simulink model "rst_auto_reg_coupled_tanks_2018b"  (R2018b)
settings: Solver=ode45  StartTime=0.0  StopTime=1000  RelTol=1e-3
InitFcn:
  | g = 981
  | Km = 3.3
  | Ao1 = 0.17
  | At1 = 15.5528
  | Ao2 = 0.17
  | At2 = 15.5528
  | Ta = 0.1
  | Ts = 50
  | ep = 0.7
libraries: dspinverses x2
settings Model: Creator=root  LastModifiedBy=root
settings DataIOCC: SaveFormat=StructureWithTime
settings OptimizationCC: LifeSpan=inf
settings DebuggingCC: LibraryContextMissingDiagnostic=none  SFExecutionAtInitializationDiag=none
settings HardwareCC: ProdBitPerSizeT=32  ProdBitPerPtrDiffT=32  ProdWordSize=32  ProdHWDeviceType=Specified
settings CodeAppCC: StateflowObjectComments=on

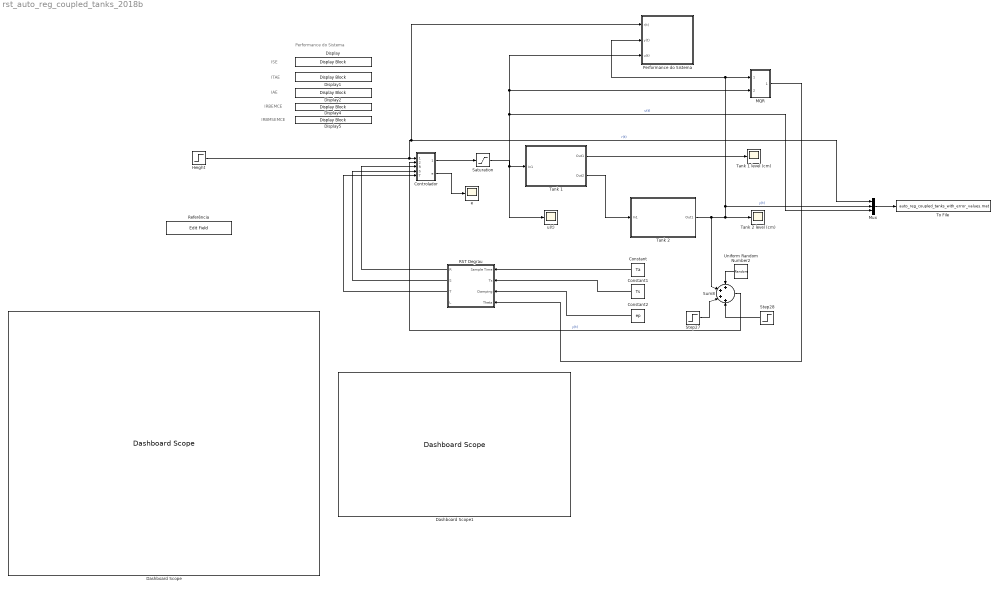
== system rst_auto_reg_coupled_tanks_2018b ==
  note: IAE
  note: IRBEMCE
  note: ISE
  note: ITAE
  note: IRBMSEMCE
  note: Performance do Sistema
  Constant : Constant  Value=Ta
  Constant1 : Constant  Value=Ts
  Constant2 : Constant  Value=ep
  Controlador : Subsystem
  Dashboard Scope : DashboardScope  WebBlockId=688
  Dashboard Scope1 : DashboardScope  WebBlockId=689
  Display : DisplayBlock  WebBlockId=787  LabelPosition=Hide
  Display1 : DisplayBlock  WebBlockId=788  LabelPosition=Hide
  Display2 : DisplayBlock  WebBlockId=789  LabelPosition=Hide
  Display4 : DisplayBlock  WebBlockId=790  LabelPosition=Hide
  Display5 : DisplayBlock  WebBlockId=791  LabelPosition=Hide
  Height : Step  Time=0  After=15  SampleTime=0
  MQR : Subsystem
  Mux : Mux  Inputs=3
  Performance do Sistema : Subsystem
  RST Degrau : Subsystem
  Referência : EditField  WebBlockId=683  LabelPosition=Hide  Alignment=Center
  Saturation : Saturate  UpperLimit=12  LowerLimit=-12
  Step27 : Step  Time=150  SampleTime=0
  Step28 : Step  Time=151  After=-1  SampleTime=0
  Sum8 : Sum  Inputs=++++
  Tank 1 : Subsystem
  "Tank 1 level (cm) " : Scope
  Tank 2 : Subsystem
  "Tank 2 level (cm) " : Scope
  To File : ToFile  Filename=auto_reg_coupled_tanks_with_error_values.mat
  Uniform Random Number2 : UniformRandomNumber  Minimum=-0.01  Maximum=0.01  SampleTime=0
  e : Scope
  u(t) : Scope
  wires:
  Constant2/1 -> RST Degrau/3(Damping)
  Constant/1 -> RST Degrau/1(Sample Time)
  Constant1/1 -> RST Degrau/2(Ts)
  MQR/1("Theta(t) ") -> RST Degrau/4(Theta)
  Tank 1/1(Out1) -> "Tank 1 level (cm) "/1
  Tank 1/2(Out2) -> Tank 2/1(In1)
  RST Degrau/1(R) -> Controlador/3(R)
  RST Degrau/2(S) -> Controlador/4(S)
  RST Degrau/3(T) -> Controlador/5(T)
  Controlador/1(u(t)) -> Saturation/1
  Controlador/2("e ") -> e/1
  Step27/1 -> Sum8/3
  Step28/1 -> Sum8/4
  Uniform Random Number2/1 -> Sum8/1
  Sum8/1 -> Controlador/2(y(t))  "y(t)"
  Mux/1 -> To File/1
  Saturation/1 -> u(t)/1, Mux/3, Performance do Sistema/3(u(t)), MQR/2("u(t) "), Tank 1/1(In1)  "u(t)"
  Tank 2/1(Out1) -> Sum8/2, Mux/2, Performance do Sistema/2(y(t)), MQR/1(y(t)), "Tank 2 level (cm) "/1  "y(t)"
  Height/1 -> Performance do Sistema/1(r(t)), Mux/1, Controlador/1(r(t))  "r(t)"

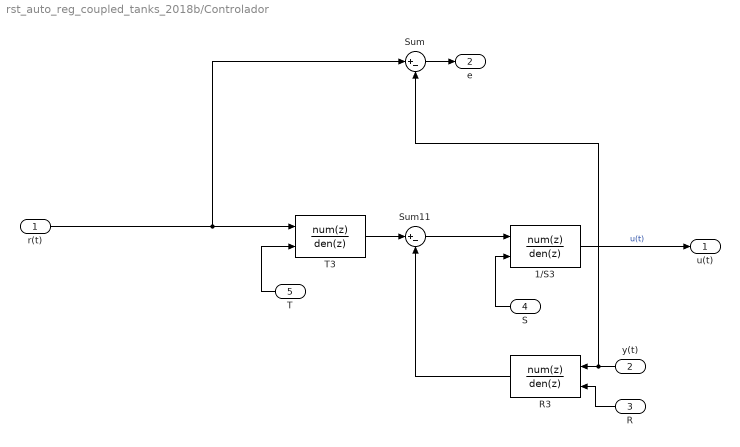
== system rst_auto_reg_coupled_tanks_2018b/Controlador ==
  r(t) : Inport
  y(t) : Inport  Port=2
  R : Inport  Port=3
  S : Inport  Port=4
  T : Inport  Port=5
  1/S3 : DiscreteFilter  Numerator=1  DenominatorSource=Input port  Denominator=1  SampleTime=Ta  a0EqualsOne=on
      settings: InputPortMap=u0,p3
  R3 : DiscreteFilter  NumeratorSource=Input port  Numerator=[-620.2 131.3]  Denominator=1  SampleTime=Ta
      settings: InputPortMap=u0,p1
  Sum : Sum  Inputs=|+-
  Sum11 : Sum  Inputs=|+-
  T3 : DiscreteFilter  NumeratorSource=Input port  Numerator=13.39  Denominator=1  SampleTime=Ta
      settings: InputPortMap=u0,p1
  u(t) : Outport
  "e " : Outport  Port=2
  wires:
  R/1 -> R3/2
  R3/1 -> Sum11/2
  Sum11/1 -> 1/S3/1
  T3/1 -> Sum11/1
  y(t)/1 -> Sum/2, R3/1
  S/1 -> 1/S3/2
  r(t)/1 -> Sum/1, T3/1
  T/1 -> T3/2
  1/S3/1 -> u(t)/1  "u(t)"
  Sum/1 -> "e "/1

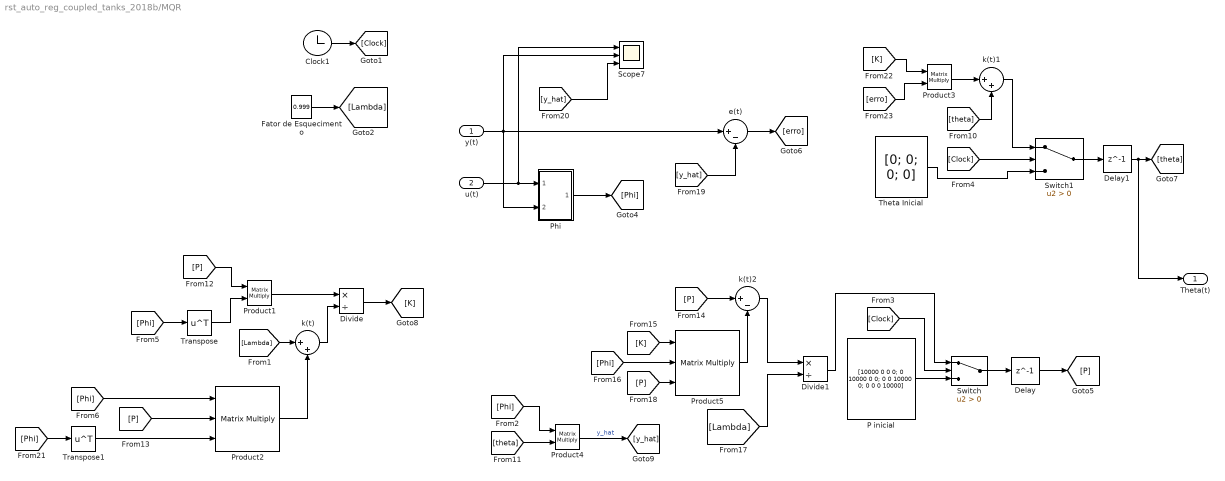
== system rst_auto_reg_coupled_tanks_2018b/MQR ==
  y(t) : Inport
  "u(t) " : Inport  Port=2
  Clock1 : Clock
  Delay : Delay  DelayLength=1  InitialCondition=0
  Delay1 : Delay  DelayLength=1  InitialCondition=0
  Divide : Product  Inputs=*/
  Divide1 : Product  Inputs=*/
  "Fator de Esquecimento " : Constant  Value=0.999
  P inicial : Constant  Value=[10000 0 0 0; 0 10000 0 0; 0 0 10000 0; 0 0 0 10000]
  Phi : Subsystem
  Product1 : Product  Multiplication=Matrix(*)
  Product2 : Product  Inputs=3  Multiplication=Matrix(*)
  Product3 : Product  Multiplication=Matrix(*)
  Product4 : Product  Multiplication=Matrix(*)
  Product5 : Product  Inputs=3  Multiplication=Matrix(*)
  Scope7 : Scope  NumInputPorts=3
  Switch : Switch  Criteria=u2 > Threshold
  Switch1 : Switch  Criteria=u2 > Threshold
  "Theta Inicial " : Constant  Value=[0; 0; 0; 0]
  Transpose : Math  Operator=transpose  SaturateOnIntegerOverflow=on
  Transpose1 : Math  Operator=transpose  SaturateOnIntegerOverflow=on
  e(t) : Sum  Inputs=|+-
  k(t) : Sum  Inputs=|++
  k(t)1 : Sum  Inputs=|++
  k(t)2 : Sum  Inputs=|+-
  "Theta(t) " : Outport
  wires:
  k(t)/1 -> Divide/2
  [Phi] -> Product4/1
  Phi/1(Phi) -> [Phi]
  k(t)1/1 -> Switch1/1
  [y_hat] -> Scope7/3
  Switch1/1 -> Delay1/1
  [K] -> Product3/1
  Product2/1 -> k(t)/2
  [Clock] -> Switch1/2
  y(t)/1 -> e(t)/1, Scope7/2, Phi/2(y(t))
  k(t)2/1 -> Divide1/1
  Delay1/1 -> "Theta(t) "/1, [theta]
  Product5/1 -> k(t)2/2
  "u(t) "/1 -> Scope7/1, Phi/1(u(t))
  Switch/1 -> Delay/1
  [Lambda] -> Divide1/2
  Product1/1 -> Divide/1
  e(t)/1 -> [erro]
  Product3/1 -> k(t)1/1
  Delay/1 -> [P]
  [Phi] -> Transpose1/1
  [P] -> Product5/3
  "Fator de Esquecimento "/1 -> [Lambda]
  "Theta Inicial "/1 -> Switch1/3
  Transpose1/1 -> Product2/3
  Divide1/1 -> Switch/1
  [Phi] -> Transpose/1
  [Clock] -> Switch/2
  [theta] -> Product4/2
  [P] -> k(t)2/1
  [theta] -> k(t)1/2
  [P] -> Product2/2
  [Lambda] -> k(t)/1
  Transpose/1 -> Product1/2
  Clock1/1 -> [Clock]
  [erro] -> Product3/2
  [y_hat] -> e(t)/2
  [K] -> Product5/1
  P inicial/1 -> Switch/3
  [P] -> Product1/1
  [Phi] -> Product2/1
  Divide/1 -> [K]
  [Phi] -> Product5/2
  Product4/1 -> [y_hat]  "y_hat"

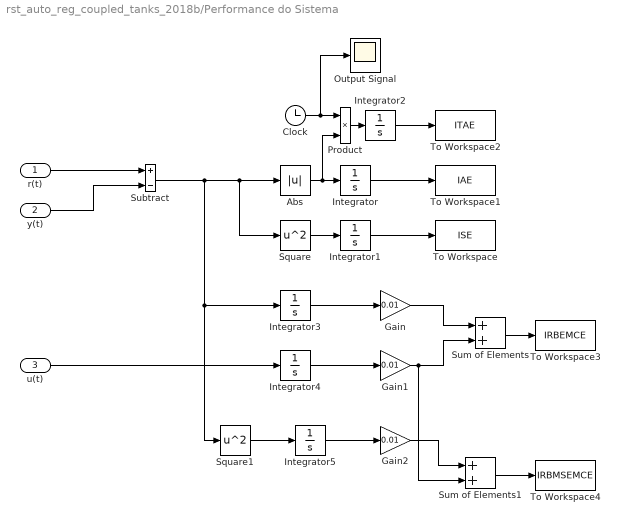
== system rst_auto_reg_coupled_tanks_2018b/Performance do Sistema ==
  r(t) : Inport
  y(t) : Inport  Port=2
  u(t) : Inport  Port=3
  Abs : Abs
  Clock : Clock
  Gain : Gain  Gain=0.01
  Gain1 : Gain  Gain=0.01
  Gain2 : Gain  Gain=0.01
  Integrator{,1..5} (6 alike) : Integrator
  Output Signal : Scope
  Product : Product
  Square : Math  Operator=square  SaturateOnIntegerOverflow=on
  Square1 : Math  Operator=square  SaturateOnIntegerOverflow=on
  Subtract : Sum  Inputs=+-
  Sum of Elements : Sum
  Sum of Elements1 : Sum
  To Workspace : ToWorkspace  VariableName=ISE  SaveFormat=Timeseries  SampleTime=-1
  To Workspace1 : ToWorkspace  VariableName=IAE  SaveFormat=Timeseries  SampleTime=-1
  To Workspace2 : ToWorkspace  VariableName=ITAE  SaveFormat=Timeseries  SampleTime=-1
  To Workspace3 : ToWorkspace  VariableName=IRBEMCE  SaveFormat=Timeseries  SampleTime=-1
  To Workspace4 : ToWorkspace  VariableName=IRBMSEMCE  SaveFormat=Timeseries  SampleTime=-1
  wires:
  y(t)/1 -> Subtract/2
  Abs/1 -> Product/2, Integrator/1
  Integrator/1 -> To Workspace1/1
  Integrator1/1 -> To Workspace/1
  Square/1 -> Integrator1/1
  Clock/1 -> Output Signal/1, Product/1
  Product/1 -> Integrator2/1
  Integrator2/1 -> To Workspace2/1
  r(t)/1 -> Subtract/1
  Subtract/1 -> Square1/1, Integrator3/1, Square/1, Abs/1
  Integrator3/1 -> Gain/1
  Integrator4/1 -> Gain1/1
  Gain/1 -> Sum of Elements/1
  Gain1/1 -> Sum of Elements1/2, Sum of Elements/2
  Square1/1 -> Integrator5/1
  Integrator5/1 -> Gain2/1
  Gain2/1 -> Sum of Elements1/1
  Sum of Elements/1 -> To Workspace3/1
  Sum of Elements1/1 -> To Workspace4/1
  u(t)/1 -> Integrator4/1

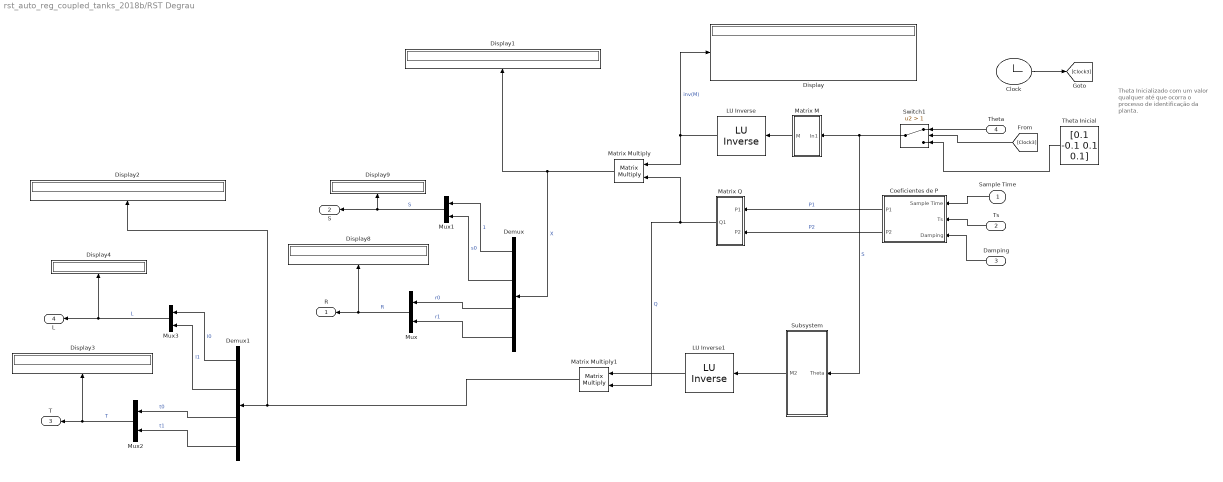
== system rst_auto_reg_coupled_tanks_2018b/RST Degrau ==
  note: Theta Inicializado com um
      | valor qualquer até que ocorra
      |  o processo de identificação
      | da planta.
  Sample Time : Inport
  Ts : Inport  Port=2
  Damping : Inport  Port=3
  Theta : Inport  Port=4
  " LU Inverse" : dspinverses/ LU Inverse
      settings: SourceProductName=DSP System Toolbox
  " LU Inverse1" : dspinverses/ LU Inverse
      settings: SourceProductName=DSP System Toolbox
  Clock : Clock
  Coeficientes de P : Subsystem
  Demux : Demux
  Demux1 : Demux
  Display{,1..4,8..9} (7 alike) : Display
  Matrix M : Subsystem
  Matrix Multiply : Product  Multiplication=Matrix(*)
  Matrix Multiply1 : Product  Multiplication=Matrix(*)
  Matrix Q : Subsystem
  Mux{,1..3} (4 alike) : Mux  Inputs=2
  Subsystem : Subsystem
  Switch1 : Switch  Criteria=u2 > Threshold  Threshold=1
  Theta Inicial : Constant  Value=[0.1 -0.1 0.1 0.1]
  R : Outport
  S : Outport  Port=2
  T : Outport  Port=3
  L : Outport  Port=4
  wires:
  Matrix Multiply/1 -> Demux/1, Display1/1  "X"
  " LU Inverse"/1 -> Matrix Multiply/1, Display/1  "inv(M)"
  Mux1/1 -> S/1, Display9/1  "S"
  Coeficientes de P/2(P2) -> Matrix Q/2(P2)  "P2"
  Ts/1 -> Coeficientes de P/2(Ts)
  Damping/1 -> Coeficientes de P/3(Damping)
  Sample Time/1 -> Coeficientes de P/1(Sample Time)
  Coeficientes de P/1(P1) -> Matrix Q/1(P1)  "P1"
  Mux/1 -> R/1, Display8/1  "R"
  Clock/1 -> [Clock3]
  Switch1/1 -> Subsystem/1(Theta), Matrix M/1(In1)  "S"
  Theta/1 -> Switch1/1
  [Clock3] -> Switch1/2
  Theta Inicial/1 -> Switch1/3
  Matrix M/1(M) -> " LU Inverse"/1
  Demux/1 -> Mux1/1  "1"
  Demux/2 -> Mux1/2  "s0"
  Demux/3 -> Mux/1  "r0"
  Demux/4 -> Mux/2  "r1"
  " LU Inverse1"/1 -> Matrix Multiply1/1
  Matrix Q/1(Q1) -> Matrix Multiply1/2, Matrix Multiply/2  "Q"
  Subsystem/1(M2) -> " LU Inverse1"/1
  Demux1/3 -> Mux2/1  "t0"
  Mux2/1 -> T/1, Display3/1  "T"
  Demux1/2 -> Mux3/2  "l1"
  Mux3/1 -> L/1, Display4/1  "L"
  Demux1/1 -> Mux3/1  "l0"
  Matrix Multiply1/1 -> Display2/1, Demux1/1
  Demux1/4 -> Mux2/2  "t1"

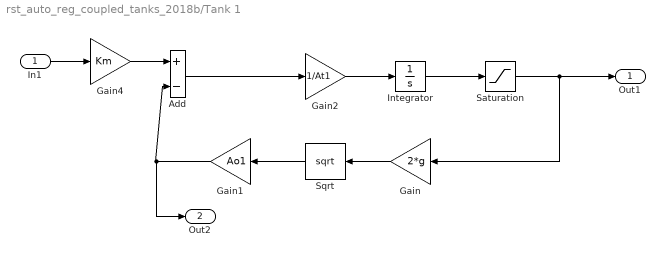
== system rst_auto_reg_coupled_tanks_2018b/Tank 1 ==
  In1 : Inport
  Add : Sum  Inputs=+-
  Gain : Gain  Gain=2*g
  Gain1 : Gain  Gain=Ao1
  Gain2 : Gain  Gain=1/At1
  Gain4 : Gain  Gain=Km
  Integrator : Integrator
  Saturation : Saturate  UpperLimit=30  LowerLimit=0
  Sqrt : Sqrt  SaturateOnIntegerOverflow=on
  Out1 : Outport
  Out2 : Outport  Port=2
  wires:
  Gain2/1 -> Integrator/1
  Gain1/1 -> Out2/1, Add/2
  Gain/1 -> Sqrt/1
  In1/1 -> Gain4/1
  Sqrt/1 -> Gain1/1
  Integrator/1 -> Saturation/1
  Saturation/1 -> Out1/1, Gain/1
  Add/1 -> Gain2/1
  Gain4/1 -> Add/1

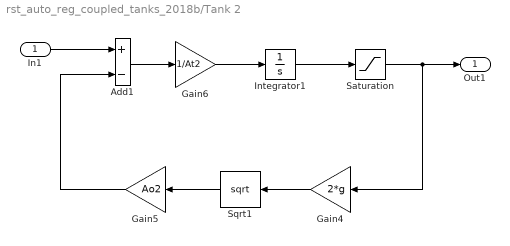
== system rst_auto_reg_coupled_tanks_2018b/Tank 2 ==
  In1 : Inport
  Add1 : Sum  Inputs=+-
  Gain4 : Gain  Gain=2*g
  Gain5 : Gain  Gain=Ao2
  Gain6 : Gain  Gain=1/At2
  Integrator1 : Integrator
  Saturation : Saturate  UpperLimit=30  LowerLimit=0
  Sqrt1 : Sqrt  SaturateOnIntegerOverflow=on
  Out1 : Outport
  wires:
  Add1/1 -> Gain6/1
  Gain6/1 -> Integrator1/1
  In1/1 -> Add1/1
  Sqrt1/1 -> Gain5/1
  Gain4/1 -> Sqrt1/1
  Integrator1/1 -> Saturation/1
  Gain5/1 -> Add1/2
  Saturation/1 -> Out1/1, Gain4/1

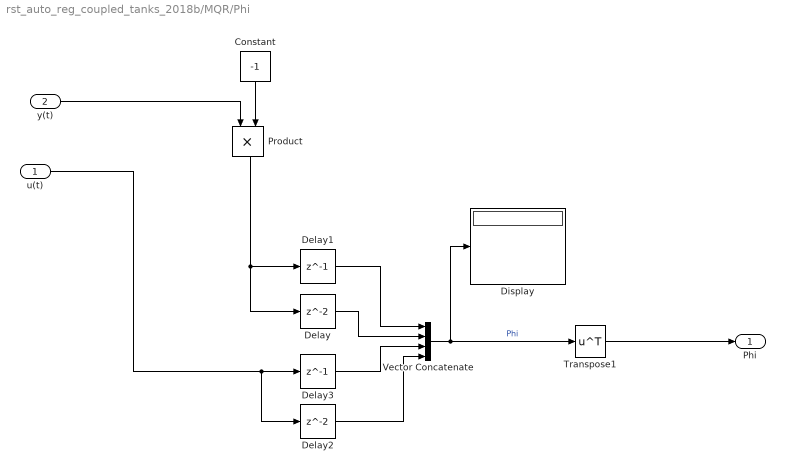
== system rst_auto_reg_coupled_tanks_2018b/MQR/Phi ==
  u(t) : Inport
  y(t) : Inport  Port=2
  Constant : Constant  Value=-1
  Delay : Delay
  Delay1 : Delay  DelayLength=1
  Delay2 : Delay
  Delay3 : Delay  DelayLength=1
  Display : Display
  Product : Product
  Transpose1 : Math  Operator=transpose  SaturateOnIntegerOverflow=on
  Vector Concatenate : Concatenate  NumInputs=4
  Phi : Outport
  wires:
  u(t)/1 -> Delay2/1, Delay3/1
  Vector Concatenate/1 -> Transpose1/1, Display/1  "Phi"
  Delay/1 -> Vector Concatenate/2
  y(t)/1 -> Product/1
  Delay3/1 -> Vector Concatenate/3
  Delay2/1 -> Vector Concatenate/4
  Delay1/1 -> Vector Concatenate/1
  Transpose1/1 -> Phi/1
  Constant/1 -> Product/2
  Product/1 -> Delay/1, Delay1/1

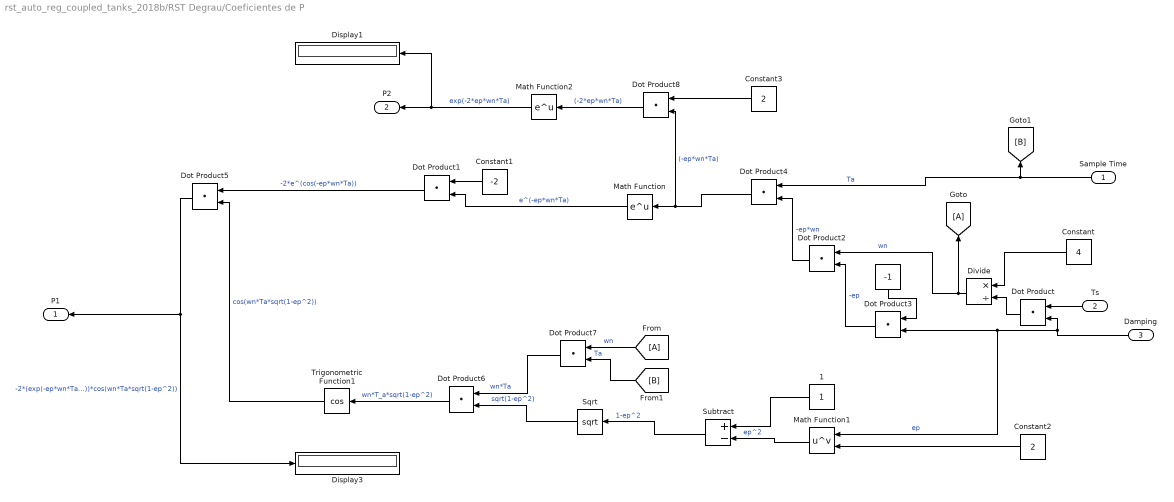
== system rst_auto_reg_coupled_tanks_2018b/RST Degrau/Coeficientes de P ==
  Sample Time : Inport
  Ts : Inport  Port=2
  Damping : Inport  Port=3
  " " : Constant  Value=-1
  1 : Constant
  Constant : Constant  Value=4
  Constant1 : Constant  Value=-2
  Constant2 : Constant  Value=2
  Constant3 : Constant  Value=2
  Display1 : Display
  Display3 : Display
  Divide : Product  Inputs=*/
  Dot Product{,1..8} (9 alike) : DotProduct  InputSameDT=on  OutDataTypeStr=Inherit: Inherit via internal rule
  Math Function : Math  SaturateOnIntegerOverflow=on
  Math Function1 : Math  Operator=pow  SaturateOnIntegerOverflow=on
  Math Function2 : Math  SaturateOnIntegerOverflow=on
  Sqrt : Sqrt  SaturateOnIntegerOverflow=on
  Subtract : Sum  Inputs=+-
  Trigonometric Function1 : Trigonometry  Operator=cos
  P1 : Outport
  P2 : Outport  Port=2
  wires:
  Math Function/1 -> Dot Product1/2  "e^(-ep*wn*Ta)"
  Divide/1 -> [A], Dot Product2/1  "wn"
  [A] -> Dot Product7/1  "wn"
  " "/1 -> Dot Product3/1
  Dot Product5/1 -> P1/1, Display3/1  "-2*(exp(-ep*wn*Ta))*cos(wn*Ta*sqrt(1-ep^2))"
  Trigonometric Function1/1 -> Dot Product5/2  "cos(wn*Ta*sqrt(1-ep^2))"
  Ts/1 -> Dot Product/1
  Dot Product/1 -> Divide/2
  Dot Product3/1 -> Dot Product2/2  "-ep"
  Damping/1 -> Math Function1/1, Dot Product3/2, Dot Product/2  "ep"
  Constant/1 -> Divide/1
  Dot Product7/1 -> Dot Product6/1  "wn*Ta"
  Sample Time/1 -> Dot Product4/1, [B]  "Ta"
  Math Function1/1 -> Subtract/2  "ep^2"
  Dot Product1/1 -> Dot Product5/1  "-2*e^(cos(-ep*wn*Ta))"
  Constant2/1 -> Math Function1/2
  1/1 -> Subtract/1
  Constant1/1 -> Dot Product1/1
  Dot Product2/1 -> Dot Product4/2  "-ep*wn"
  [B] -> Dot Product7/2  "Ta"
  Dot Product6/1 -> Trigonometric Function1/1  "wn*T_a*sqrt(1-ep^2)"
  Dot Product4/1 -> Dot Product8/2, Math Function/1  "(-ep*wn*Ta)"
  Sqrt/1 -> Dot Product6/2  "sqrt(1-ep^2)"
  Subtract/1 -> Sqrt/1  "1-ep^2"
  Constant3/1 -> Dot Product8/1
  Dot Product8/1 -> Math Function2/1  "(-2*ep*wn*Ta)"
  Math Function2/1 -> Display1/1, P2/1  "exp(-2*ep*wn*Ta)"

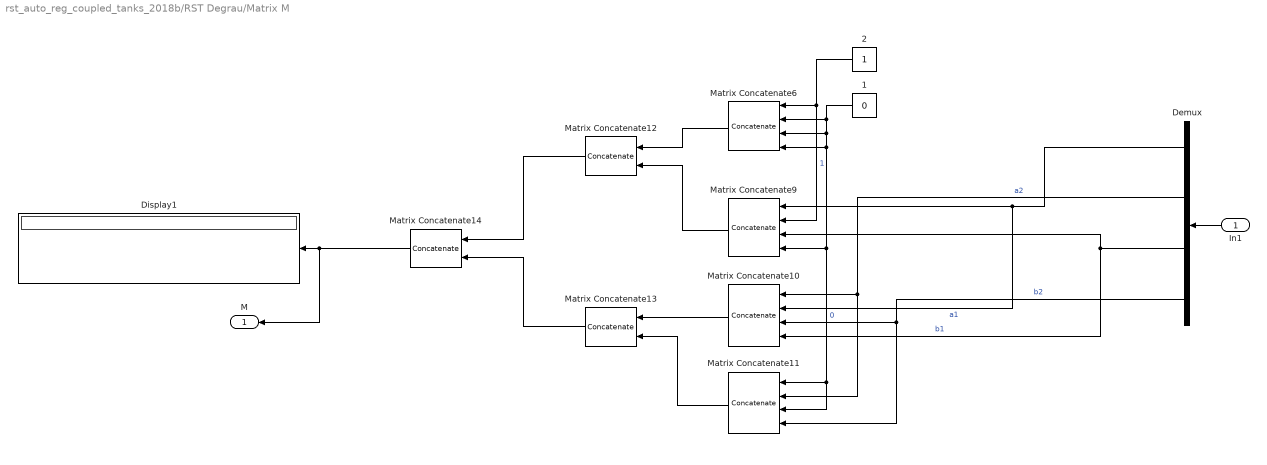
== system rst_auto_reg_coupled_tanks_2018b/RST Degrau/Matrix M ==
  In1 : Inport
  " 1" : Constant  Value=0
  2 : Constant
  Demux : Demux
  Display1 : Display
  Matrix Concatenate{6,9..11} (4 alike) : Concatenate  NumInputs=4  Mode=Multidimensional array  ConcatenateDimension=2
  Matrix Concatenate12 : Concatenate  Mode=Multidimensional array
  Matrix Concatenate13 : Concatenate  Mode=Multidimensional array
  Matrix Concatenate14 : Concatenate  Mode=Multidimensional array
  M : Outport
  wires:
  In1/1 -> Demux/1
  Demux/3 -> Matrix Concatenate9/3, Matrix Concatenate10/4  "b1"
  Matrix Concatenate14/1 -> M/1, Display1/1
  Demux/1 -> Matrix Concatenate10/2, Matrix Concatenate9/1  "a1"
  Demux/4 -> Matrix Concatenate11/4, Matrix Concatenate10/3  "b2"
  Demux/2 -> Matrix Concatenate11/2, Matrix Concatenate10/1  "a2"
  2/1 -> Matrix Concatenate9/2, Matrix Concatenate6/1  "1"
  " 1"/1 -> Matrix Concatenate6/3, Matrix Concatenate11/3, Matrix Concatenate11/1, Matrix Concatenate9/4, Matrix Concatenate6/4, Matrix Concatenate6/2  "0"
  Matrix Concatenate6/1 -> Matrix Concatenate12/1
  Matrix Concatenate9/1 -> Matrix Concatenate12/2
  Matrix Concatenate10/1 -> Matrix Concatenate13/1
  Matrix Concatenate11/1 -> Matrix Concatenate13/2
  Matrix Concatenate13/1 -> Matrix Concatenate14/2
  Matrix Concatenate12/1 -> Matrix Concatenate14/1

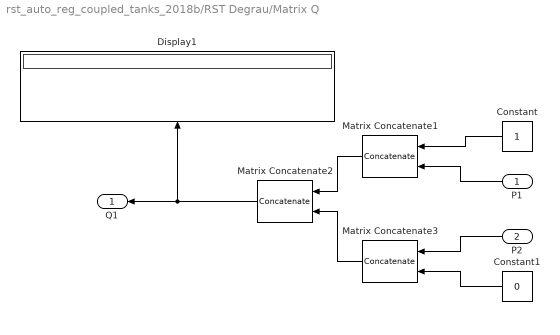
== system rst_auto_reg_coupled_tanks_2018b/RST Degrau/Matrix Q ==
  P1 : Inport
  P2 : Inport  Port=2
  Constant : Constant
  Constant1 : Constant  Value=0
  Display1 : Display
  Matrix Concatenate1 : Concatenate  Mode=Multidimensional array
  Matrix Concatenate2 : Concatenate  Mode=Multidimensional array
  Matrix Concatenate3 : Concatenate  Mode=Multidimensional array
  Q1 : Outport
  wires:
  Matrix Concatenate1/1 -> Matrix Concatenate2/1
  Matrix Concatenate2/1 -> Q1/1, Display1/1
  Matrix Concatenate3/1 -> Matrix Concatenate2/2
  P2/1 -> Matrix Concatenate3/1
  P1/1 -> Matrix Concatenate1/2
  Constant/1 -> Matrix Concatenate1/1
  Constant1/1 -> Matrix Concatenate3/2

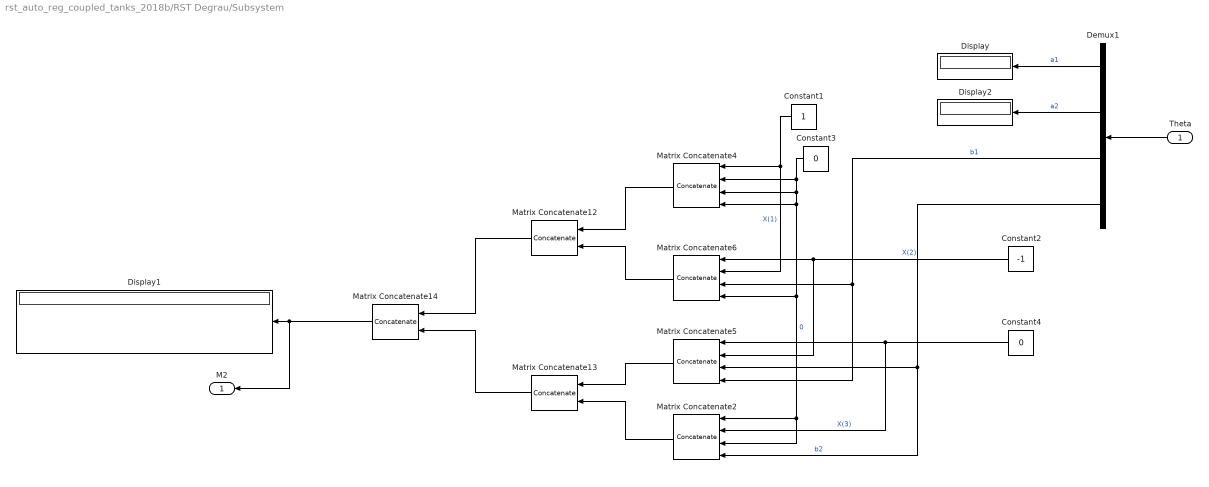
== system rst_auto_reg_coupled_tanks_2018b/RST Degrau/Subsystem ==
  Theta : Inport
  Constant1 : Constant
  Constant2 : Constant  Value=-1
  Constant3 : Constant  Value=0
  Constant4 : Constant  Value=0
  Demux1 : Demux
  Display : Display
  Display1 : Display
  Display2 : Display
  Matrix Concatenate12 : Concatenate  Mode=Multidimensional array
  Matrix Concatenate13 : Concatenate  Mode=Multidimensional array
  Matrix Concatenate14 : Concatenate  Mode=Multidimensional array
  Matrix Concatenate{2,4..6} (4 alike) : Concatenate  NumInputs=4  Mode=Multidimensional array  ConcatenateDimension=2
  M2 : Outport
  wires:
  Matrix Concatenate6/1 -> Matrix Concatenate12/2
  Demux1/2 -> Display2/1  "a2"
  Theta/1 -> Demux1/1
  Demux1/1 -> Display/1  "a1"
  Constant1/1 -> Matrix Concatenate6/2, Matrix Concatenate4/1  "X(1)"
  Constant3/1 -> Matrix Concatenate4/3, Matrix Concatenate2/3, Matrix Concatenate2/1, Matrix Concatenate6/4, Matrix Concatenate4/4, Matrix Concatenate4/2  "0"
  Demux1/3 -> Matrix Concatenate5/4, Matrix Concatenate6/3  "b1"
  Demux1/4 -> Matrix Concatenate2/4, Matrix Concatenate5/3  "b2"
  Matrix Concatenate14/1 -> Display1/1, M2/1
  Matrix Concatenate13/1 -> Matrix Concatenate14/2
  Matrix Concatenate12/1 -> Matrix Concatenate14/1
  Matrix Concatenate4/1 -> Matrix Concatenate12/1
  Matrix Concatenate5/1 -> Matrix Concatenate13/1
  Matrix Concatenate2/1 -> Matrix Concatenate13/2
  Constant2/1 -> Matrix Concatenate5/2, Matrix Concatenate6/1  "X(2)"
  Constant4/1 -> Matrix Concatenate2/2, Matrix Concatenate5/1  "X(3)"
